simulink model "cav_adas_mpc"  (R2022a)
settings: Solver=VariableStepAuto  StartTime=0.0  StopTime=500  RelTol=1e-2
values from neighbouring files (symbols this model uses):
  Af = 2.33    [data_cav.m]
  Cd = 0.28    [data_cav.m]
  elev_date_1 = date_elev(:,1)    [data_cav.m]
  elev_date_2 = date_elev(:,2)    [data_cav.m]
  eta = 0.93    [data_cav.m]
  fr = 0.015    [data_cav.m]
  g = 9.81    [data_cav.m]
  m = 1521    [data_cav.m]
  R = 0.5    [data_cav.m]
  rho = 1.2    [data_cav.m]
  slope_date_1 = date_slope(:,1)    [data_cav.m]
  slope_date_2_degree = zeros(length(slope_date_2_grad),1)    [data_cav.m]
undefined symbols (not defined in the file or in its folder): sigbuilder_block
libraries: mpclib x1
settings Model: Creator=user  LastModifiedBy=user

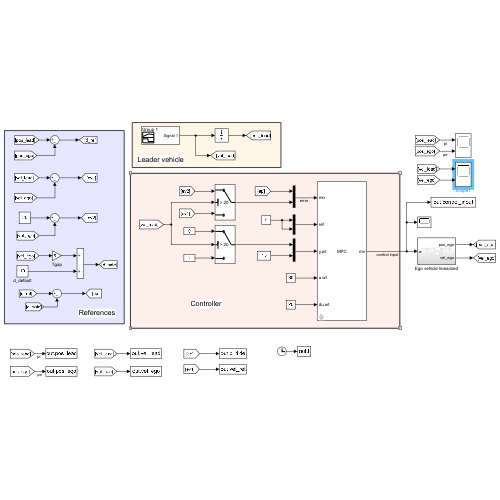
[thumbnail: Simulink's stored preview of the top-level diagram]
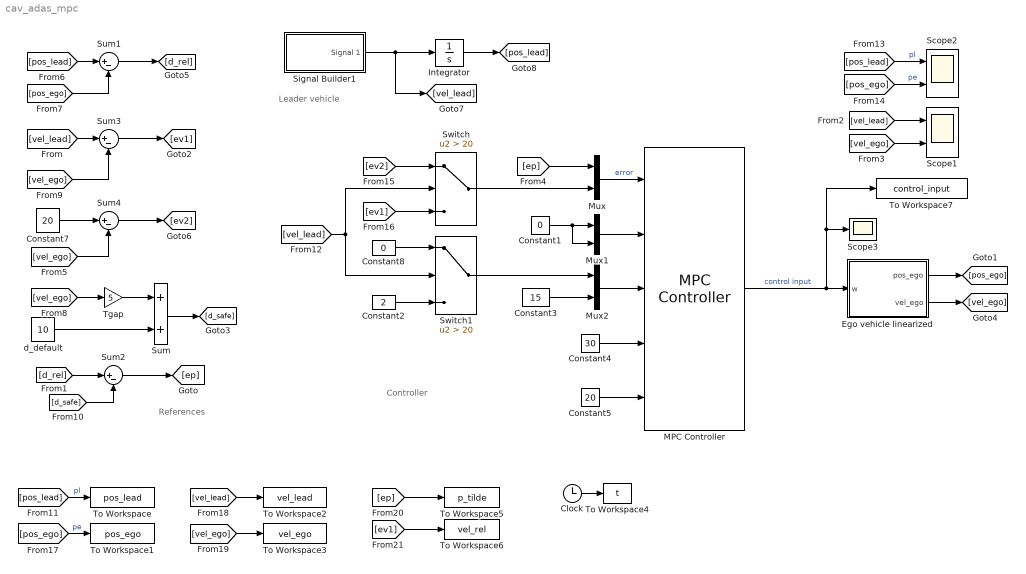
== system cav_adas_mpc ==
  note: Controller
  note: References
  note: Leader vehicle
  Clock : Clock
  Constant1 : Constant  Value=0
  Constant2 : Constant  Value=2
  Constant3 : Constant  Value=15
  Constant4 : Constant  Value=30
  Constant5 : Constant  Value=20
  Constant7 : Constant  Value=20
  Constant8 : Constant  Value=0
  Ego vehicle linearized : Subsystem
  Integrator : Integrator  InitialCondition=30
  MPC Controller : mpclib/MPC Controller  SCDEnableBlockLinearizationSpecification=on  mpcobj=mpc1  is_multiple=0  enable_value=0  return_u0=off  updateMPCinCallerWorkspace=on  md_inport=off  mv_inport=off  uref_inport=off  return_cost=off  return_mvseq=off  return_qpstatus=off  return_xseq=off  return_state=off  return_ovseq=off  state_inport=off  umin_inport=off  umax_inport=off  ymin_inport=off  ymax_inport=off  cc_inport=off  ywt_inport=on  uwt_inport=on  duwt_inport=on  rhoeps_inport=off  pm_inport=off  MaximumP=10  HorizonChoice=FixedHorizon  n_ts=0.1  n_p=50  n_mv=1  n_md=0  n_ud=0  n_mo=2  n_uo=0  BlockDataType=double  SampleTimeInherited=off  switch_inport=off
  Mux : Mux  Inputs=2
  Mux1 : Mux  Inputs=2
  Mux2 : Mux  Inputs=2
  Scope1 : Scope  NumInputPorts=2
  Scope2 : Scope  NumInputPorts=2
  Scope3 : Scope
  Signal Builder1 : Subsystem  Tag=STV Subsys  LoadFcn=sigbuilder_block('load');  StartFcn=sigbuilder_block('start');  StopFcn=sigbuilder_block('stop');  ClipboardFcn=sigbuilder_block('clipboard');  mask(Sigbuilder block){tuvar=[0:10]}
      mask help: Simulink:masks:SigbuilderBlock_MD
      mask init:
      | if ~strcmp(get_param(bdroot(gcbh),'SimulationStatus'),'stopped') tuvar = sigbuilder_block('maskInit'); end
      settings: CopyFcn=sigbuilder_block('copy');  DeleteFcn=sigbuilder_block('delete');  ModelCloseFcn=sigbuilder_block('modelClose');  PreSaveFcn=sigbuilder_block('preSave');  PauseFcn=sigbuilder_block('pause');  ContinueFcn=sigbuilder_block('continue');  NameChangeFcn=sigbuilder_block('namechange');  OpenFcn=sigbuilder_block('open',[391.2 97.2 550.8 400.2 ]);  CloseFcn=sigbuilder_block('close');
      mask Display: plot(0, 0, 100, 100,[2, 2, 32, 32, 2], [68, 8, 8, 68, 68],[32, 2], [38, 38], [32, 19, 2],[53, 60, 44], [32, 17, 17, 2],[16, 16, 31, 31]);txt = getActiveGroup(gcbh);text(2, 100, txt,'verticalAlignment', 'top');
  Sum : Sum
  Sum{1..4} (4 alike) : Sum  Inputs=|+-
  Switch : Switch  Criteria=u2 > Threshold  Threshold=20  SaturateOnIntegerOverflow=off  InputSameDT=off
  Switch1 : Switch  Criteria=u2 > Threshold  Threshold=20  SaturateOnIntegerOverflow=off  InputSameDT=off
  Tgap : Gain  Gain=5
  To Workspace : ToWorkspace  VariableName=pos_lead  SampleTime=-1
      settings: Save2DSignal=2-D array (concatenate along first dimension)
  To Workspace1 : ToWorkspace  VariableName=pos_ego  SampleTime=-1
      settings: Save2DSignal=2-D array (concatenate along first dimension)
  To Workspace2 : ToWorkspace  VariableName=vel_lead  SampleTime=-1
      settings: Save2DSignal=2-D array (concatenate along first dimension)
  To Workspace3 : ToWorkspace  VariableName=vel_ego  SampleTime=-1
      settings: Save2DSignal=2-D array (concatenate along first dimension)
  To Workspace4 : ToWorkspace  VariableName=t  SampleTime=-1
      settings: Save2DSignal=2-D array (concatenate along first dimension)
  To Workspace5 : ToWorkspace  VariableName=p_tilde  SampleTime=-1
      settings: Save2DSignal=2-D array (concatenate along first dimension)
  To Workspace6 : ToWorkspace  VariableName=vel_rel  SampleTime=-1
      settings: Save2DSignal=2-D array (concatenate along first dimension)
  To Workspace7 : ToWorkspace  VariableName=control_input  SampleTime=-1
      settings: Save2DSignal=2-D array (concatenate along first dimension)
  d_default : Constant  Value=10
  wires:
  Integrator/1 -> [pos_lead]
  Signal Builder1/1(Signal 1) -> [vel_lead], Integrator/1
  [pos_lead] -> Scope2/1  "pl"
  [pos_ego] -> Scope2/2  "pe"
  [vel_lead] -> Scope1/1
  [vel_ego] -> Scope1/2
  [pos_lead] -> Sum1/1
  [pos_ego] -> Sum1/2
  Sum1/1 -> [d_rel]
  Sum3/1 -> [ev1]
  [vel_lead] -> Sum3/1
  [vel_ego] -> Sum3/2
  MPC Controller/1 -> To Workspace7/1, Scope3/1, Ego vehicle linearized/1(w)  "control input"
  Mux/1 -> MPC Controller/1  "error"
  Mux1/1 -> MPC Controller/2
  Constant1/1 -> Mux1/2, Mux1/1
  Sum2/1 -> [ep]
  [ep] -> Mux/1
  Mux2/1 -> MPC Controller/3
  Constant3/1 -> Mux2/2
  Constant4/1 -> MPC Controller/4
  Constant5/1 -> MPC Controller/5
  Tgap/1 -> Sum/1
  [vel_ego] -> Tgap/1
  Sum/1 -> [d_safe]
  d_default/1 -> Sum/2
  Sum4/1 -> [ev2]
  [vel_lead] -> Switch1/2, Switch/2
  Constant2/1 -> Switch1/3
  [ev1] -> Switch/3
  [ev2] -> Switch/1
  Constant8/1 -> Switch1/1
  Switch/1 -> Mux/2
  Switch1/1 -> Mux2/1
  Constant7/1 -> Sum4/1
  [vel_ego] -> Sum4/2
  [d_safe] -> Sum2/2
  [d_rel] -> Sum2/1
  Ego vehicle linearized/1(pos_ego) -> [pos_ego]
  Ego vehicle linearized/2(vel_ego) -> [vel_ego]
  [pos_lead] -> To Workspace/1  "pl"
  [pos_ego] -> To Workspace1/1  "pe"
  [vel_lead] -> To Workspace2/1
  [vel_ego] -> To Workspace3/1
  Clock/1 -> To Workspace4/1
  [ev1] -> To Workspace6/1
  [ep] -> To Workspace5/1

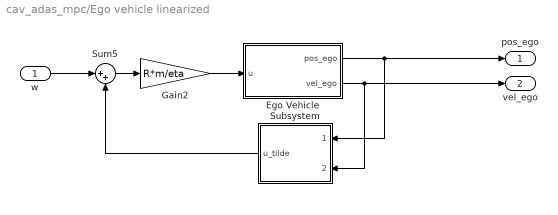
== system cav_adas_mpc/Ego vehicle linearized ==
  w : Inport
  "Ego Vehicle " : Subsystem
  Gain2 : Gain  Gain=R*m/eta
  Subsystem : Subsystem
  Sum5 : Sum  Inputs=|++
  pos_ego : Outport
  vel_ego : Outport  Port=2
  wires:
  "Ego Vehicle "/2(vel_ego) -> vel_ego/1, Subsystem/2(vel_ego)
  "Ego Vehicle "/1(pos_ego) -> pos_ego/1, Subsystem/1(pos_ego)
  Sum5/1 -> Gain2/1
  w/1 -> Sum5/1
  Gain2/1 -> "Ego Vehicle "/1(u)
  Subsystem/1(u_tilde) -> Sum5/2

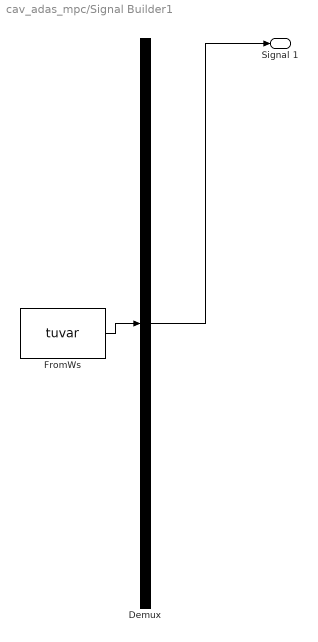
== system cav_adas_mpc/Signal Builder1 ==
  Demux : Demux  Tag=STV Demux  Outputs=1
      settings: DisplayOption=none
  FromWs : FromWorkspace  Tag=STV FromWs  VariableName=tuvar
      SigBuilderData=|
      | common.afterFinalStr = 'Extrapolate'
      | common.sampleTime = 0
      | dataSet.timeRange = [0 400]
      | dataSet.name = 'Group 1'
      | sbobj.Groups.Name = 'Group 1'
      | sbobj.Groups.Signals.Name = 'Signal 1'
      | sbobj.Groups.Signals.XData = [0 75 75 150 150 200 200 275 275 350 350 400]
      | sbobj.Groups.Signals.YData = [18 18 10 10 20 20 15 15 5 5 0 0]
      | sbobj.Groups.TimeRange = [0 400]
  Signal 1 : Outport  Tag=STV Outport
  wires:
  FromWs/1 -> Demux/1
  Demux/1 -> Signal 1/1

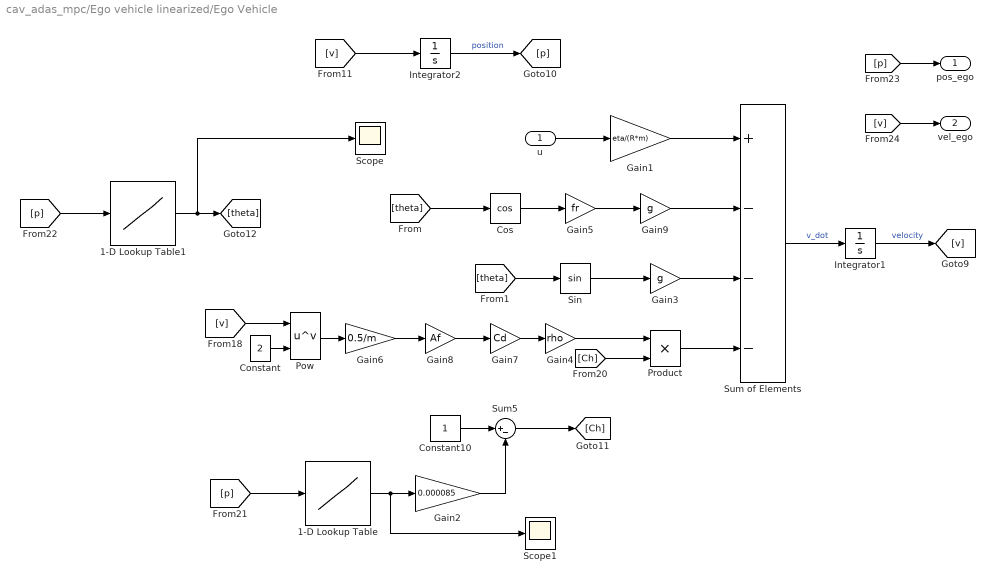
== system cav_adas_mpc/Ego vehicle linearized/Ego Vehicle  ==
  u : Inport
  1-D Lookup Table : Lookup_n-D  NumberOfTableDimensions=1  BreakpointsForDimension1=elev_date_1  Table=elev_date_2  InternalRulePriority=Speed  RndMeth=Simplest
  1-D Lookup Table1 : Lookup_n-D  NumberOfTableDimensions=1  BreakpointsForDimension1=slope_date_1  Table=slope_date_2_degree  InternalRulePriority=Speed  RndMeth=Simplest
  Constant : Constant  Value=2
  Constant10 : Constant
  Cos : Trigonometry  Operator=cos
  Gain1 : Gain  Gain=eta/(R*m)
  Gain2 : Gain  Gain=0.000085
  Gain3 : Gain  Gain=g
  Gain4 : Gain  Gain=rho
  Gain5 : Gain  Gain=fr
  Gain6 : Gain  Gain=0.5/m
  Gain7 : Gain  Gain=Cd
  Gain8 : Gain  Gain=Af
  Gain9 : Gain  Gain=g
  Integrator1 : Integrator
  Integrator2 : Integrator
  Pow : Math  Operator=pow  RndMeth=Zero
  Product : Product
  Scope : Scope
  Scope1 : Scope
  Sin : Trigonometry
  Sum of Elements : Sum  Inputs=+---
  Sum5 : Sum  Inputs=|+-
  pos_ego : Outport
  vel_ego : Outport  Port=2
  wires:
  [p] -> 1-D Lookup Table/1
  1-D Lookup Table1/1 -> Scope/1, [theta]
  Gain5/1 -> Gain9/1
  Gain6/1 -> Gain8/1
  [Ch] -> Product/2
  Sin/1 -> Gain3/1
  Gain4/1 -> Product/1
  Sum5/1 -> [Ch]
  Gain1/1 -> Sum of Elements/1
  Integrator2/1 -> [p]  "position"
  Constant10/1 -> Sum5/1
  Gain9/1 -> Sum of Elements/2
  Integrator1/1 -> [v]  "velocity"
  Pow/1 -> Gain6/1
  Gain8/1 -> Gain7/1
  Gain2/1 -> Sum5/2
  Cos/1 -> Gain5/1
  Sum of Elements/1 -> Integrator1/1  "v_dot"
  1-D Lookup Table/1 -> Scope1/1, Gain2/1
  Gain7/1 -> Gain4/1
  [v] -> vel_ego/1
  [v] -> Integrator2/1
  Constant/1 -> Pow/2
  [p] -> 1-D Lookup Table1/1
  [v] -> Pow/1
  Gain3/1 -> Sum of Elements/3
  [p] -> pos_ego/1
  Product/1 -> Sum of Elements/4
  u/1 -> Gain1/1
  [theta] -> Cos/1
  [theta] -> Sin/1

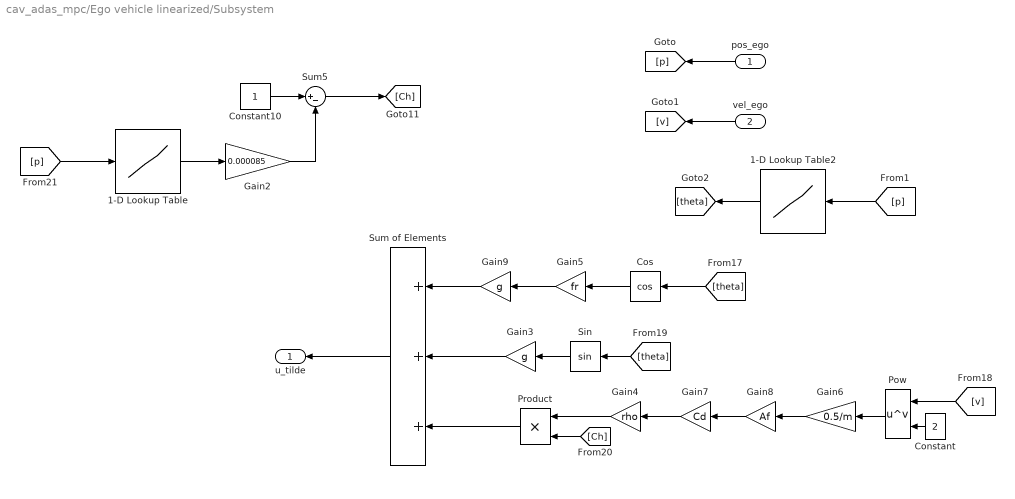
== system cav_adas_mpc/Ego vehicle linearized/Subsystem ==
  pos_ego : Inport
  vel_ego : Inport  Port=2
  1-D Lookup Table : Lookup_n-D  NumberOfTableDimensions=1  BreakpointsForDimension1=elev_date_1  Table=elev_date_2  InternalRulePriority=Speed  RndMeth=Simplest
  1-D Lookup Table2 : Lookup_n-D  NumberOfTableDimensions=1  BreakpointsForDimension1=slope_date_1  Table=slope_date_2_degree  InternalRulePriority=Speed  RndMeth=Simplest
  Constant : Constant  Value=2
  Constant10 : Constant
  Cos : Trigonometry  Operator=cos
  Gain2 : Gain  Gain=0.000085
  Gain3 : Gain  Gain=g
  Gain4 : Gain  Gain=rho
  Gain5 : Gain  Gain=fr
  Gain6 : Gain  Gain=0.5/m
  Gain7 : Gain  Gain=Cd
  Gain8 : Gain  Gain=Af
  Gain9 : Gain  Gain=g
  Pow : Math  Operator=pow  RndMeth=Zero
  Product : Product
  Sin : Trigonometry
  Sum of Elements : Sum  Inputs=+++
  Sum5 : Sum  Inputs=|+-
  u_tilde : Outport
  wires:
  pos_ego/1 -> [p]
  vel_ego/1 -> [v]
  Cos/1 -> Gain5/1
  Sin/1 -> Gain3/1
  Gain7/1 -> Gain4/1
  [v] -> Pow/1
  Gain8/1 -> Gain7/1
  Gain6/1 -> Gain8/1
  Constant/1 -> Pow/2
  Pow/1 -> Gain6/1
  Gain4/1 -> Product/1
  [Ch] -> Product/2
  [theta] -> Sin/1
  Gain5/1 -> Gain9/1
  [p] -> 1-D Lookup Table2/1
  1-D Lookup Table2/1 -> [theta]
  1-D Lookup Table/1 -> Gain2/1
  Gain2/1 -> Sum5/2
  [p] -> 1-D Lookup Table/1
  Constant10/1 -> Sum5/1
  Sum5/1 -> [Ch]
  Sum of Elements/1 -> u_tilde/1
  [theta] -> Cos/1
  Gain9/1 -> Sum of Elements/1
  Gain3/1 -> Sum of Elements/2
  Product/1 -> Sum of Elements/3
